simulink model "dry_test"  (R2020a)
settings: Solver=FixedStepAuto  StartTime=0.0  StopTime=30  FixedStep=.1  RelTol=1e-3
libraries: robotlib x2
settings Model: EnablePacing=on  Creator=lamarre  LastModifiedBy=lamarre
settings OptimizationCC: EnhancedBackFolding=on  PassReuseOutputArgsAs=Individual arguments  ZeroExternalMemoryAtStartup=off  ZeroInternalMemoryAtStartup=off  MaxStackSize=64  OptimizeBlockOrder=speed  DifferentSizesBufferReuse=on  OptimizationCustomize=off  EfficientTunableParamExpr=on
settings DebuggingCC: ParameterTunabilityLossMsg=error
settings HardwareCC: ProdBitPerPointer=32  ProdBitPerSizeT=32  ProdBitPerPtrDiffT=32  ProdLargestAtomicInteger=Long  ProdWordSize=32  ProdHWDeviceType=ARM Compatible->ARM 8  TargetBitPerLong=64  TargetBitPerPointer=64  TargetBitPerSizeT=64  TargetBitPerPtrDiffT=64  TargetLongLongMode=on  TargetIntDivRoundTo=Zero  TargetEndianess=LittleEndian  TargetWordSize=64  TargetHWDeviceType=Custom Processor->MATLAB Host Computer  ProdEqTarget=off
settings SFSimCC: MATLABDynamicMemAlloc=off
settings RTWCC: SystemTargetFile=ert.tlc  HardwareBoard=Robot Operating System (ROS)  TemplateMakefile=ert_default_tmf  Toolchain=Catkin  TargetLang=C++
settings CodeAppCC: ForceParamTrailComments=on  IgnoreCustomStorageClasses=off  OperatorAnnotations=on  SimulinkDataObjDesc=on  SFDataObjDesc=on  InsertBlockDesc=on
settings ERTTargetCC: SupportContinuousTime=on  SupportNonInlinedSFcns=on

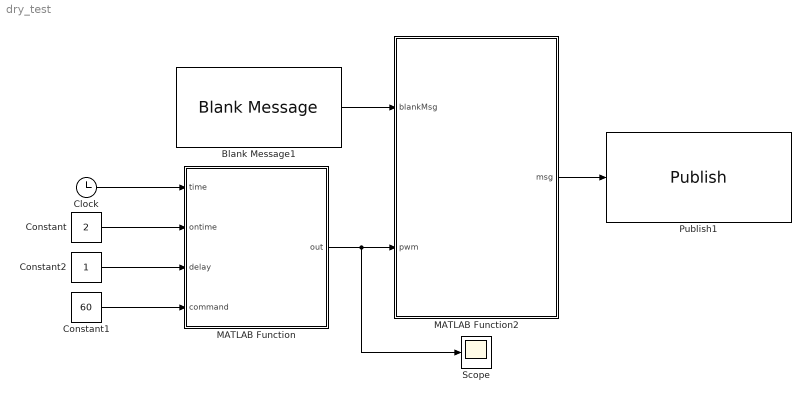
== system dry_test ==
  Blank Message1 : robotlib/Blank Message  messageClass=Message  entityType=std_msgs/UInt16MultiArray  messageType=std_msgs/UInt16MultiArray  SampleTime=inf
  Clock : Clock
  Constant : Constant  Value=2
  Constant1 : Constant  Value=60
  Constant2 : Constant
  MATLAB Function : MATLAB Function  TreatAsAtomicUnit=on
  MATLAB Function2 : MATLAB Function  TreatAsAtomicUnit=on
  Publish1 : robotlib/Publish  topicSource=Specify your own  topic=/provider_thruster/thruster_pwm  messageType=std_msgs/UInt16MultiArray  messageQueueLength=1
  Scope : Scope
  wires:
  Constant/1 -> MATLAB Function/2(ontime)
  Clock/1 -> MATLAB Function/1(time)
  Constant1/1 -> MATLAB Function/4(command)
  Constant2/1 -> MATLAB Function/3(delay)
  MATLAB Function2/1(msg) -> Publish1/1
  MATLAB Function/1(out) -> MATLAB Function2/2(pwm), Scope/1
  Blank Message1/1 -> MATLAB Function2/1(blankMsg)

== matlab function dry_test/MATLAB Function ==
  data: time input; out output size=8; ontime input; delay input; command input
function out = DryTest(time, ontime,delay, command)
out=repmat(1500,8,1);
for i=1:8
    if time>ontime*(i-1)+((i)*delay) && time<ontime*(i)+(i*delay)
       out(i)= out(i)+command;
    end
end

== matlab function dry_test/MATLAB Function2 ==
  data: blankMsg input; pwm input; msg output Bus: SL_Bus_dry_test_std_msgs_UInt16MultiArray
function msg = assignThrusterPwm(blankMsg, pwm)
msg = blankMsg;
msg.Data(1:8) = cast(pwm, 'uint16');
msg.Data_SL_Info.CurrentLength = uint32(8);
